simulink model "Product"  (R2017b)
settings: Solver=FixedStepDiscrete  StartTime=0.0  StopTime=10.0  FixedStep=0.200000  RelTol=1e-3
settings Model: Creator=hbourbou  LastModifiedBy=hbourbou
settings DataIOCC: SaveFormat=StructureWithTime
settings OptimizationCC: LifeSpan=inf
settings DebuggingCC: SFExecutionAtInitializationDiag=none
settings HardwareCC: ProdBitPerSizeT=32  ProdBitPerPtrDiffT=32  ProdWordSize=32  ProdHWDeviceType=Specified
settings CodeAppCC: StateflowObjectComments=on

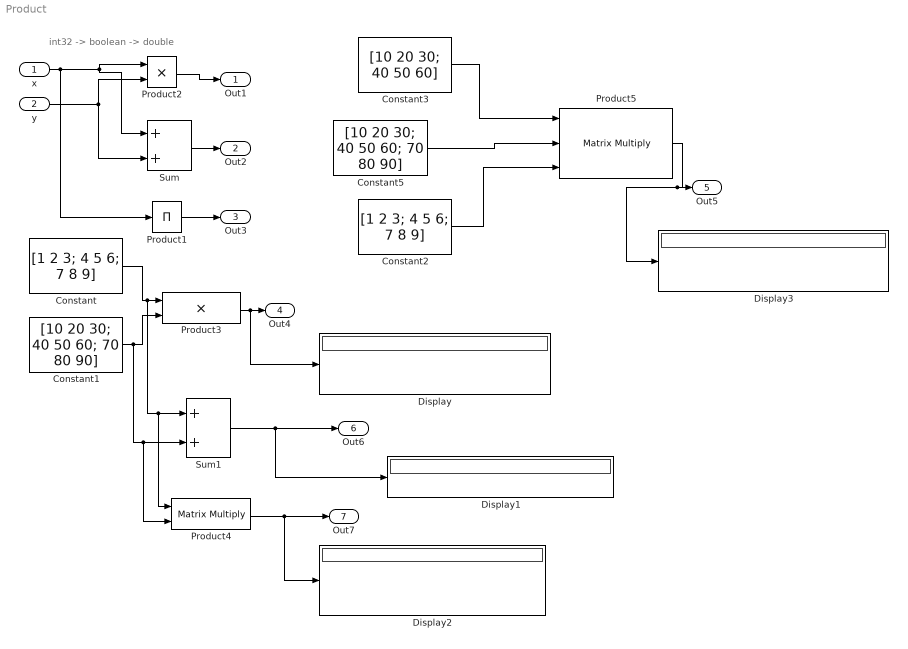
== system Product ==
  note: int32 -> boolean -> double
  x : Inport  OutDataTypeStr=uint8  PortDimensions=3
  y : Inport  Port=2  OutDataTypeStr=uint16
  Constant : Constant  Value=[1 2 3; 4 5 6; 7 8 9]
  Constant1 : Constant  Value=[10 20 30; 40 50 60; 70 80 90]
  Constant2 : Constant  Value=[1 2 3; 4 5 6; 7 8 9]
  Constant3 : Constant  Value=[10 20 30; 40 50 60]
  Constant5 : Constant  Value=[10 20 30; 40 50 60; 70 80 90]
  Display{,1..3} (4 alike) : Display
  Product1 : Product  Inputs=*
  Product2 : Product  Inputs=**
  Product3 : Product  Inputs=**
  Product4 : Product  Inputs=**  Multiplication=Matrix(*)
  Product5 : Product  Inputs=***  Multiplication=Matrix(*)
  Sum : Sum  Inputs=2
  Sum1 : Sum
  Out1 : Outport
  Out2 : Outport  Port=2
  Out3 : Outport  Port=3
  Out4 : Outport  Port=4
  Out5 : Outport  Port=5
  Out6 : Outport  Port=6
  Out7 : Outport  Port=7
  wires:
  Product2/1 -> Out1/1
  y/1 -> Product2/2, Sum/2
  Sum/1 -> Out2/1
  x/1 -> Product1/1, Sum/1, Product2/1
  Product1/1 -> Out3/1
  Constant/1 -> Product4/1, Sum1/1, Product3/1
  Constant1/1 -> Product4/2, Sum1/2, Product3/2
  Product3/1 -> Display/1, Out4/1
  Sum1/1 -> Out6/1, Display1/1
  Product4/1 -> Out7/1, Display2/1
  Constant3/1 -> Product5/1
  Product5/1 -> Display3/1, Out5/1
  Constant5/1 -> Product5/2
  Constant2/1 -> Product5/3
